simulink library "SunDirection"  (R2014b)
settings: Solver=ode45  StartTime=0.0  StopTime=10.0  RelTol=1e-3
undefined symbols (not defined in the file): ConfParam
settings Model: Creator=Hp  LastModifiedBy=Hp

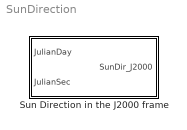
== system SunDirection ==
  Sun Direction in the J2000 frame : Subsystem

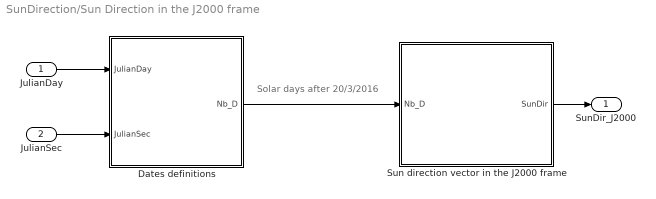
== system SunDirection/Sun Direction in the J2000 frame ==
  note: Solar days after 20/3/2016
  JulianDay : Inport
  JulianSec : Inport  Port=2
  Dates definitions : Subsystem
  Sun direction vector in the J2000 frame : Subsystem
  SunDir_J2000 : Outport
  wires:
  Sun direction vector in the J2000 frame/1(SunDir) -> SunDir_J2000/1
  Dates definitions/1(Nb_D) -> Sun direction vector in the J2000 frame/1(Nb_D)
  JulianDay/1 -> Dates definitions/1(JulianDay)
  JulianSec/1 -> Dates definitions/2(JulianSec)

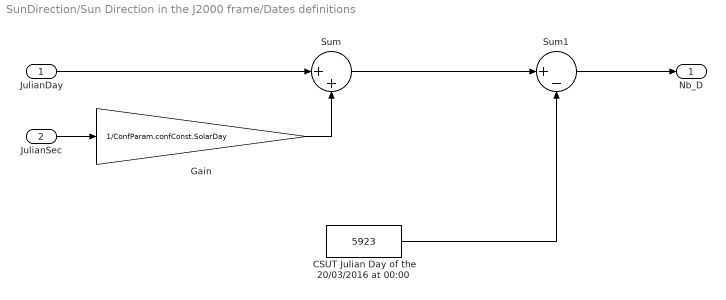
== system SunDirection/Sun Direction in the J2000 frame/Dates definitions ==
  JulianDay : Inport
  JulianSec : Inport  Port=2
  CSUT Julian Day of the 20/03/2016 at 00:00 : Constant  Value=5923
  Gain : Gain  Gain=1/ConfParam.confConst.SolarDay
  Sum : Sum  Inputs=|++
  Sum1 : Sum  Inputs=|+-
  Nb_D : Outport
  wires:
  CSUT Julian Day of the 20/03/2016 at 00:00/1 -> Sum1/2
  JulianSec/1 -> Gain/1
  Gain/1 -> Sum/2
  Sum/1 -> Sum1/1
  Sum1/1 -> Nb_D/1
  JulianDay/1 -> Sum/1

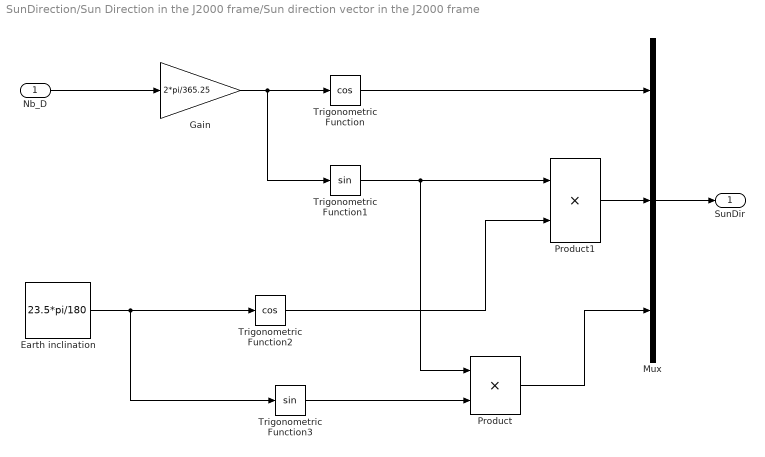
== system SunDirection/Sun Direction in the J2000 frame/Sun direction vector in the J2000 frame ==
  Nb_D : Inport
  Earth inclination : Constant  Value=23.5*pi/180
  Gain : Gain  Gain=2*pi/365.25
  Mux : Mux  Inputs=3
  Product : Product  Inputs=**
  Product1 : Product  Inputs=**
  Trigonometric Function : Trigonometry  Operator=cos
  Trigonometric Function1 : Trigonometry
  Trigonometric Function2 : Trigonometry  Operator=cos
  Trigonometric Function3 : Trigonometry
  SunDir : Outport
  wires:
  Trigonometric Function/1 -> Mux/1
  Product/1 -> Mux/3
  Mux/1 -> SunDir/1
  Trigonometric Function3/1 -> Product/2
  Product1/1 -> Mux/2
  Gain/1 -> Trigonometric Function/1, Trigonometric Function1/1
  Trigonometric Function1/1 -> Product/1, Product1/1
  Trigonometric Function2/1 -> Product1/2
  Nb_D/1 -> Gain/1
  Earth inclination/1 -> Trigonometric Function2/1, Trigonometric Function3/1
